simulink model "qr_vert_ctrl"  (R2018b)
settings: Solver=VariableStepAuto  StartTime=0.0  StopTime=30  RelTol=1e-3
PreLoadFcn:
  | load vars.mat
values from neighbouring files (symbols this model uses):
  ddz_ref = 0    [vars.mat]
  init =     [vars.mat]
  ks_pos = [1 0 0.1]    [vars.mat]
  ks_vel = [10 10 0]    [vars.mat]
  par =     [vars.mat]
  sam_tim =     [vars.mat]
  Ta = 0.1    [vars.mat]
  Tv = 0.05    [vars.mat]
  z_ref = 0.5    [vars.mat]
undefined symbols (not defined in the file or in its folder): sgn
libraries: simulink x9
settings Model: Creator=amatusv  LastModifiedBy=amatusv

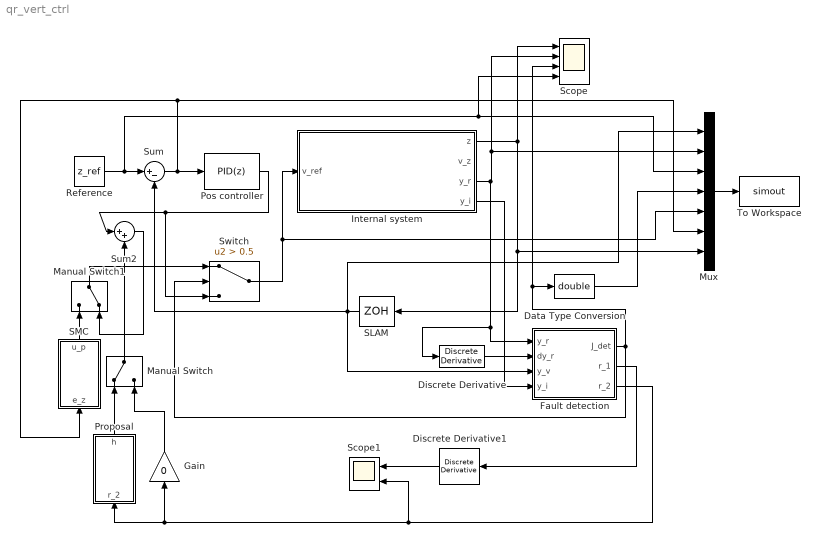
== system qr_vert_ctrl ==
  Data Type Conversion : DataTypeConversion  OutDataTypeStr=double
  Discrete Derivative : simulink/Discrete/Discrete Derivative  gainval=1.0  ICPrevScaledInput=init.z/sam_tim.bebop  OutMin=[]  OutMax=[]  OutDataType=fixdt(1, 16)  OutScaling=2^-10  DoSatur=off
  Discrete Derivative1 : simulink/Discrete/Discrete Derivative  gainval=1.0  ICPrevScaledInput=0  OutMin=[]  OutMax=[]  OutDataType=fixdt(1, 16)  OutScaling=2^-10  DoSatur=off
  Fault detection : Subsystem
  Gain : Gain  Gain=0
  Internal system : Subsystem
  Manual Switch : ManualSwitch
  Manual Switch1 : ManualSwitch  CurrentSetting=0
  Mux : Mux  Inputs=7
  Pos controller : simulink/Continuous/PID Controller  Controller=PID  Form=Parallel  TimeDomain=Discrete-time  SampleTime=-1  IntegratorMethod=Forward Euler  FilterMethod=Forward Euler  ControllerParametersSource=internal  P=ks_pos(1)  I=ks_pos(2)  D=ks_pos(3)  UseFilter=off  N=100  TunerSelectOption=Transfer Function Based (PID Tuner App)  InitialConditionSource=internal  InitialConditionForIntegrator=0  InitialConditionForFilter=0  DifferentiatorICPrevScaledInput=(z_ref - init.z)/Tv*ks_pos(3)  ExternalReset=none  TrackingMode=off  Kt=1  LimitOutput=off  UpperSaturationLimit=4.905  LowerSaturationLimit=-4.905  LinearizeAsGain=on  AntiWindupMode=none  Kb=1  POutMin=[]  POutMax=[]  IOutMin=[]  IOutMax=[]  DOutMin=[]  DOutMax=[]  NOutMin=[]  NOutMax=[]  SumOutMin=[]  SumOutMax=[]  SaturationOutMin=[]  SaturationOutMax=[]  PParamMin=[]  PParamMax=[]  IParamMin=[]  IParamMax=[]  DParamMin=[]  DParamMax=[]  NParamMin=[]  NParamMax=[]  KbParamMin=[]  KbParamMax=[]  KtParamMin=[]  KtParamMax=[]  KbOutMin=[]  KbOutMax=[]  KtOutMin=[]  KtOutMax=[]  IntegratorOutMin=[]  IntegratorOutMax=[]  FilterOutMin=[]  FilterOutMax=[]  SumI1OutMin=[]  SumI1OutMax=[]  SumI2OutMin=[]  SumI2OutMax=[]  SumI3OutMin=[]  SumI3OutMax=[]  SumI4OutMin=[]  SumI4OutMax=[]  SumDOutMin=[]  SumDOutMax=[]  DifferentiatorOutMin=[]  DifferentiatorOutMax=[]  FilterDiffOutCoefMin=[]  FilterDiffOutCoefMax=[]  ReciprocalOutMin=[]  ReciprocalOutMax=[]  SumDenOutMin=[]  SumDenOutMax=[]  SumNumOutMin=[]  SumNumOutMax=[]  DivideOutMin=[]  DivideOutMax=[]  IntegratorContinuousStateAttributes=''  IntegratorStateMustResolveToSignalObject=off  IntegratorRTWStateStorageClass=Auto  FilterContinuousStateAttributes=''  FilterStateMustResolveToSignalObject=off  FilterRTWStateStorageClass=Auto  ParallelPVariant=InternalParameters  IdealPVariant=Disabled  IVariant=InternalParameters  DVariant=InternalParameters  IntegratorVariant=Discrete  SatVariant=Disabled  AWVariant=Passthrough  PCopyVariant=Disabled  TRVariant=Disabled  FdbkBlocksVariant=Forward  IdealPFdbkVariant=Disabled  SatFdbkVariant=Disabled  DerivativeFilterVariant=Differentiator  NVariant=Passthrough  NCopyVariant=Disabled_SignalSpec  FilterICVariant=InternalICsDifferentiator  IntegratorICVariant=InternalICs  ExternalResetVariant=Disabled  TRSumVariant=Passthrough  SumFdbkVariant=Disabled  SumVariant=Sum_PID
  Proposal : Subsystem
  Reference : Constant  Value=z_ref
  SLAM : ZeroOrderHold  SampleTime=sam_tim.slam
  SMC : Subsystem
  Scope : Scope  NumInputPorts=4
  Scope1 : Scope  NumInputPorts=2
  Sum : Sum  Inputs=|+-
  Sum2 : Sum  Inputs=|++
  Switch : Switch  Criteria=u2 > Threshold  Threshold=0.5
  To Workspace : ToWorkspace  VariableName=simout  SaveFormat=Timeseries  SampleTime=-1
  wires:
  Reference/1 -> Mux/3, Scope/4, Sum/1
  Sum/1 -> Pos controller/1, SMC/1(e_z), Mux/6
  Internal system/1(z) -> Scope/1, Mux/7, SLAM/1
  Internal system/3(y_r) -> Fault detection/1(y_r), Discrete Derivative/1, Scope/2, Mux/2
  Fault detection/1(J_det) -> Data Type Conversion/1, Scope/3, Switch/2
  Switch/1 -> Internal system/1(v_ref), Mux/5
  Pos controller/1 -> Sum2/1, Switch/3
  Proposal/1(h) -> Manual Switch/1
  Manual Switch/1 -> Sum2/2
  Gain/1 -> Manual Switch/2
  SLAM/1 -> Mux/1, Sum/2, Fault detection/3(y_v)
  Discrete Derivative/1 -> Fault detection/2(dy_r)
  Internal system/4(y_i) -> Fault detection/4(y_i)
  Fault detection/2(r_1) -> Discrete Derivative1/1
  Discrete Derivative1/1 -> Scope1/1
  Fault detection/3(r_2) -> Scope1/2, Proposal/1(r_2), Gain/1
  Mux/1 -> To Workspace/1
  Data Type Conversion/1 -> Mux/4
  Sum2/1 -> Manual Switch1/2
  Manual Switch1/1 -> Switch/1
  SMC/1(u_p) -> Manual Switch1/1

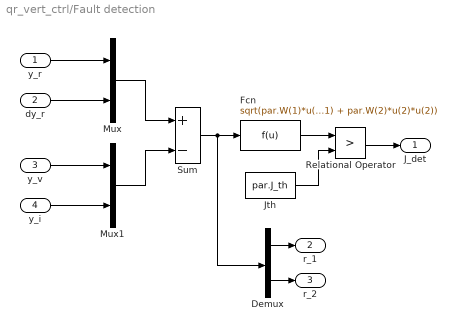
== system qr_vert_ctrl/Fault detection ==
  y_r : Inport
  dy_r : Inport  Port=2
  y_v : Inport  Port=3
  y_i : Inport  Port=4
  Demux : Demux  Outputs=2
  Fcn : Fcn  Expr=sqrt(par.W(1)*u(1)*u(1) + par.W(2)*u(2)*u(2))
  Jth : Constant  Value=par.J_th
  Mux : Mux  Inputs=2
  Mux1 : Mux  Inputs=2
  Relational Operator : RelationalOperator  Operator=>  OutDataTypeStr=boolean  RndMeth=Simplest
  Sum : Sum  Inputs=+-
  J_det : Outport
  r_1 : Outport  Port=2
  r_2 : Outport  Port=3
  wires:
  y_r/1 -> Mux/1
  dy_r/1 -> Mux/2
  y_v/1 -> Mux1/1
  y_i/1 -> Mux1/2
  Mux/1 -> Sum/1
  Mux1/1 -> Sum/2
  Sum/1 -> Demux/1, Fcn/1
  Fcn/1 -> Relational Operator/1
  Jth/1 -> Relational Operator/2
  Relational Operator/1 -> J_det/1
  Demux/1 -> r_1/1
  Demux/2 -> r_2/1

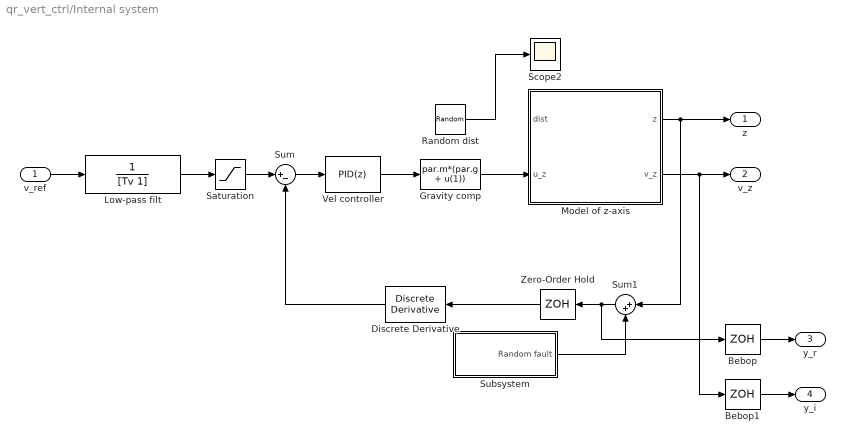
== system qr_vert_ctrl/Internal system ==
  v_ref : Inport
  Bebop : ZeroOrderHold  SampleTime=sam_tim.bebop
  Bebop1 : ZeroOrderHold  SampleTime=sam_tim.bebop
  Discrete Derivative : simulink/Discrete/Discrete Derivative  gainval=1.0  ICPrevScaledInput=init.z/sam_tim.inner  OutMin=[]  OutMax=[]  OutDataType=fixdt(1, 16)  OutScaling=2^-10  DoSatur=off
  Gravity comp : Fcn  Expr=par.m*(par.g + u(1))
  Low-pass filt : TransferFcn  Denominator=[Tv 1]
  Model of z-axis : Subsystem
  Random dist : RandomNumber  Variance=0.01  SampleTime=0.1
  Saturation : Saturate  UpperLimit=1.0  LowerLimit=-1.0  ZeroCross=off
  Scope2 : Scope
  Subsystem : Subsystem
  Sum : Sum  Inputs=|+-
  Sum1 : Sum  Inputs=|++
  Vel controller : simulink/Continuous/PID Controller  Controller=PID  Form=Parallel  TimeDomain=Discrete-time  SampleTime=-1  IntegratorMethod=Forward Euler  FilterMethod=Forward Euler  ControllerParametersSource=internal  P=ks_vel(1)  I=ks_vel(2)  D=ks_vel(3)  UseFilter=off  N=100  TunerSelectOption=Transfer Function Based (PID Tuner App)  InitialConditionSource=internal  InitialConditionForIntegrator=0  InitialConditionForFilter=0  DifferentiatorICPrevScaledInput=0  ExternalReset=none  TrackingMode=off  Kt=1  LimitOutput=on  UpperSaturationLimit=par.g/2  LowerSaturationLimit=-par.g/2  LinearizeAsGain=on  AntiWindupMode=none  Kb=1  POutMin=[]  POutMax=[]  IOutMin=[]  IOutMax=[]  DOutMin=[]  DOutMax=[]  NOutMin=[]  NOutMax=[]  SumOutMin=[]  SumOutMax=[]  SaturationOutMin=[]  SaturationOutMax=[]  PParamMin=[]  PParamMax=[]  IParamMin=[]  IParamMax=[]  DParamMin=[]  DParamMax=[]  NParamMin=[]  NParamMax=[]  KbParamMin=[]  KbParamMax=[]  KtParamMin=[]  KtParamMax=[]  KbOutMin=[]  KbOutMax=[]  KtOutMin=[]  KtOutMax=[]  IntegratorOutMin=[]  IntegratorOutMax=[]  FilterOutMin=[]  FilterOutMax=[]  SumI1OutMin=[]  SumI1OutMax=[]  SumI2OutMin=[]  SumI2OutMax=[]  SumI3OutMin=[]  SumI3OutMax=[]  SumI4OutMin=[]  SumI4OutMax=[]  SumDOutMin=[]  SumDOutMax=[]  DifferentiatorOutMin=[]  DifferentiatorOutMax=[]  FilterDiffOutCoefMin=[]  FilterDiffOutCoefMax=[]  ReciprocalOutMin=[]  ReciprocalOutMax=[]  SumDenOutMin=[]  SumDenOutMax=[]  SumNumOutMin=[]  SumNumOutMax=[]  DivideOutMin=[]  DivideOutMax=[]  IntegratorContinuousStateAttributes=''  IntegratorStateMustResolveToSignalObject=off  IntegratorRTWStateStorageClass=Auto  FilterContinuousStateAttributes=''  FilterStateMustResolveToSignalObject=off  FilterRTWStateStorageClass=Auto  ParallelPVariant=InternalParameters  IdealPVariant=Disabled  IVariant=InternalParameters  DVariant=InternalParameters  IntegratorVariant=Discrete  SatVariant=Enabled  AWVariant=Passthrough  PCopyVariant=Disabled  TRVariant=Disabled  FdbkBlocksVariant=Forward  IdealPFdbkVariant=Disabled  SatFdbkVariant=Disabled  DerivativeFilterVariant=Differentiator  NVariant=Passthrough  NCopyVariant=Disabled_SignalSpec  FilterICVariant=InternalICsDifferentiator  IntegratorICVariant=InternalICs  ExternalResetVariant=Disabled  TRSumVariant=Passthrough  SumFdbkVariant=Disabled  SumVariant=Sum_PID
  Zero-Order Hold : ZeroOrderHold  SampleTime=sam_tim.inner
  z : Outport
  v_z : Outport  Port=2
  y_r : Outport  Port=3
  y_i : Outport  Port=4
  wires:
  Saturation/1 -> Sum/1
  Sum/1 -> Vel controller/1
  Model of z-axis/1(z) -> z/1, Sum1/1
  Gravity comp/1 -> Model of z-axis/2(u_z)
  Random dist/1 -> Scope2/1
  Vel controller/1 -> Gravity comp/1
  Low-pass filt/1 -> Saturation/1
  v_ref/1 -> Low-pass filt/1
  Zero-Order Hold/1 -> Discrete Derivative/1
  Discrete Derivative/1 -> Sum/2
  Sum1/1 -> Bebop/1, Zero-Order Hold/1
  Bebop/1 -> y_r/1
  Model of z-axis/2(v_z) -> v_z/1, Bebop1/1
  Bebop1/1 -> y_i/1
  Subsystem/1(Random fault) -> Sum1/2

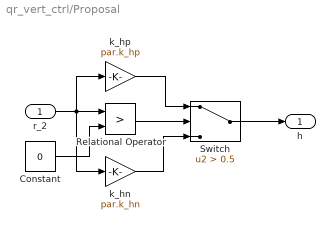
== system qr_vert_ctrl/Proposal ==
  r_2 : Inport
  Constant : Constant  Value=0
  Relational Operator : RelationalOperator  Operator=>  OutDataTypeStr=boolean  RndMeth=Simplest
  Switch : Switch  Criteria=u2 > Threshold  Threshold=0.5
  k_hn : Gain  Gain=par.k_hn
  k_hp : Gain  Gain=par.k_hp
  h : Outport
  wires:
  r_2/1 -> k_hn/1, k_hp/1, Relational Operator/1
  Constant/1 -> Relational Operator/2
  Relational Operator/1 -> Switch/2
  k_hp/1 -> Switch/1
  k_hn/1 -> Switch/3
  Switch/1 -> h/1

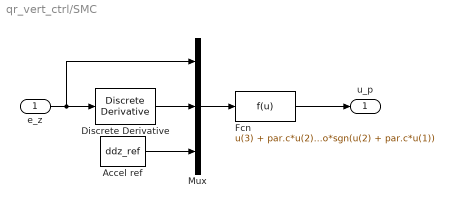
== system qr_vert_ctrl/SMC ==
  e_z : Inport
  Accel ref : Constant  Value=ddz_ref
  Discrete Derivative : simulink/Discrete/Discrete Derivative  gainval=1.0  ICPrevScaledInput=0.0  OutMin=[]  OutMax=[]  OutDataType=fixdt(1, 16)  OutScaling=2^-10  DoSatur=off
  Fcn : Fcn  Expr=u(3) + par.c*u(2) - par.rho*sgn(u(2) + par.c*u(1))
  Mux : Mux  Inputs=3
  u_p : Outport
  wires:
  e_z/1 -> Mux/1, Discrete Derivative/1
  Discrete Derivative/1 -> Mux/2
  Accel ref/1 -> Mux/3
  Mux/1 -> Fcn/1
  Fcn/1 -> u_p/1

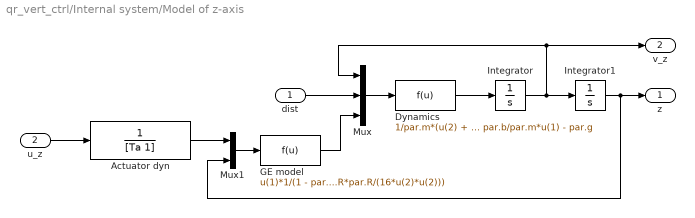
== system qr_vert_ctrl/Internal system/Model of z-axis ==
  dist : Inport
  u_z : Inport  Port=2
  Actuator dyn : TransferFcn  Denominator=[Ta 1]
  Dynamics : Fcn  Expr=1/par.m*(u(2) + u(3)) - par.b/par.m*u(1) - par.g
  GE model : Fcn  Expr=u(1)*1/(1 - par.R*par.R/(16*u(2)*u(2)))
  Integrator : Integrator  InitialCondition=init.vz
  Integrator1 : Integrator  InitialCondition=init.z
  Mux : Mux  Inputs=3
  Mux1 : Mux  Inputs=2
  z : Outport
  v_z : Outport  Port=2
  wires:
  Integrator1/1 -> Mux1/2, z/1
  Dynamics/1 -> Integrator/1
  Mux/1 -> Dynamics/1
  Integrator/1 -> v_z/1, Mux/1, Integrator1/1
  dist/1 -> Mux/2
  Mux1/1 -> GE model/1
  u_z/1 -> Actuator dyn/1
  Actuator dyn/1 -> Mux1/1
  GE model/1 -> Mux/3

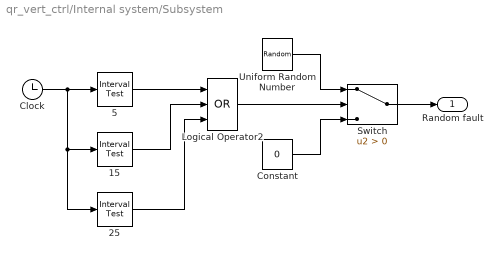
== system qr_vert_ctrl/Internal system/Subsystem ==
  15 : simulink/Logic and Bit Operations/Interval Test  IntervalClosedRight=on  uplimit=17  IntervalClosedLeft=on  lowlimit=15  OutDataTypeStr=boolean
  25 : simulink/Logic and Bit Operations/Interval Test  IntervalClosedRight=on  uplimit=28  IntervalClosedLeft=on  lowlimit=25  OutDataTypeStr=boolean
  5 : simulink/Logic and Bit Operations/Interval Test  IntervalClosedRight=on  uplimit=6  IntervalClosedLeft=on  lowlimit=5  OutDataTypeStr=boolean
  Clock : Clock
  Constant : Constant  Value=0
  Logical Operator2 : Logic  Operator=OR  Inputs=3  AllPortsSameDT=off  OutDataTypeStr=boolean
  Switch : Switch  Criteria=u2 > Threshold
  Uniform Random Number : UniformRandomNumber  Minimum=0.01  Maximum=0.2  SampleTime=sam_tim.bebop
  Random fault : Outport
  wires:
  Logical Operator2/1 -> Switch/2
  Uniform Random Number/1 -> Switch/1
  Constant/1 -> Switch/3
  Switch/1 -> Random fault/1
  Clock/1 -> 25/1, 15/1, 5/1
  5/1 -> Logical Operator2/1
  15/1 -> Logical Operator2/2
  25/1 -> Logical Operator2/3
